simulink model "my_cpm_demod_offline_model"  (R2014b)
settings: Solver=ode45  StartTime=0.0  StopTime=.4  RelTol=1e-3
undefined symbols (not defined in the file or in its folder): cpmDemodOfflineSampleTime
libraries: siglabs_lib x1
settings Model: Creator=Ben  LastModifiedBy=Ben

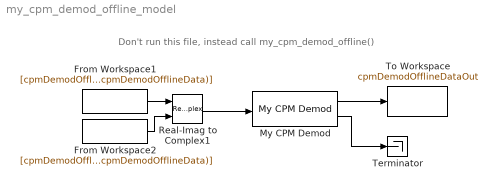
== system my_cpm_demod_offline_model ==
  note: Don't run this file, instead call my_cpm_demod_offline()
  From Workspace1 : FromWorkspace  VariableName=[cpmDemodOfflineTimeValues real(cpmDemodOfflineData)]  OutDataTypeStr=double  SampleTime=cpmDemodOfflineSampleTime  Interpolate=off  OutputAfterFinalValue=Setting to zero
  From Workspace2 : FromWorkspace  VariableName=[cpmDemodOfflineTimeValues imag(cpmDemodOfflineData)]  OutDataTypeStr=double  SampleTime=cpmDemodOfflineSampleTime  Interpolate=off  OutputAfterFinalValue=Setting to zero
  My CPM Demod : siglabs_lib/My CPM Demod  SampsPerSym=50  RotationsPerSym=1  PatternVectorDialog=[ones(1,7)*1 ones(1,7)*2 ones(1,6)*0]  PatternVectorRepeatDialog=2
  Real-Imag to Complex1 : RealImagToComplex
  Terminator : Terminator
  To Workspace : ToWorkspace  VariableName=cpmDemodOfflineDataOut  SampleTime=-1
  wires:
  From Workspace2/1 -> Real-Imag to Complex1/2
  From Workspace1/1 -> Real-Imag to Complex1/1
  Real-Imag to Complex1/1 -> My CPM Demod/1
  My CPM Demod/1 -> To Workspace/1
  My CPM Demod/2 -> Terminator/1
